simulink model "identyfikacja_zawor2_reczny"  (R2014b)
settings: Solver=ode5  StartTime=0.0  StopTime=43.6  FixedStep=0.05  RelTol=1e-3
values from neighbouring files (symbols this model uses):
  b = 40    [charakterystyki_zawory_reczne.m]    (also in daneZawory_cz2.mat; pomiary.m; rhs.m)
  c = p(1)    [cel.m]    (also in charakterystyki_zawory_reczne.m = 10; daneZawory_cz2.mat = 10; identyfikacja_parametrow.m = 10; identyfikacja_zawor2.m = 10)
  C2 = q/sqrt(H2pp)    [linearyzacja_analitycznie.m]    (also in wskaznikZawor2.m = parametry(1))
  H2max = 40    [charakterystyki_zawory_reczne.m]    (also in daneZawory_cz2.mat; pomiary.m)
  w = 5    [charakterystyka_pompa.m]    (also in charakterystyka_pompa_sterownik.m; dane14listopad.mat; danePompa.mat; pomiary.m)
  x02 = parametry(2)    [wskaznikZawor2.m]
settings Model: Creator=Michal  LastModifiedBy=Michal
settings DebuggingCC: UnderspecifiedInitializationDetection=Classic  MergeDetectMultiDrivingBlocksExec=none

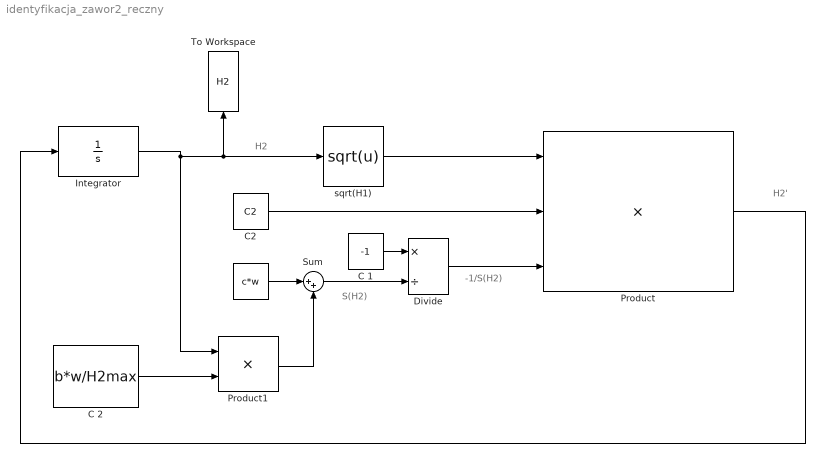
== system identyfikacja_zawor2_reczny ==
  note: -1/S(H2)
  note: S(H2)
  note: H2'
  note: H2
  " " : Constant  Value=c*w
  C 1 : Constant  Value=-1
  C 2 : Constant  Value=b*w/H2max
  "C2 " : Constant  Value=C2
  Divide : Product  Inputs=*/
  Integrator : Integrator  InitialCondition=x02
  Product : Product  Inputs=3
  Product1 : Product
  Sum : Sum  Inputs=|++
  To Workspace : ToWorkspace  VariableName=H2  SaveFormat=Structure With Time  SampleTime=-1
  sqrt(H1) : Fcn  Expr=sqrt(u)
  wires:
  Integrator/1 -> Product1/1, To Workspace/1, sqrt(H1)/1
  Product/1 -> Integrator/1
  sqrt(H1)/1 -> Product/1
  "C2 "/1 -> Product/2
  " "/1 -> Sum/1
  C 2/1 -> Product1/2
  Product1/1 -> Sum/2
  Sum/1 -> Divide/2
  C 1/1 -> Divide/1
  Divide/1 -> Product/3
